simulink model "MatlabDDE"  (Simulink 7.3)
settings: Solver=ode3  StartTime=0.0  StopTime=inf  FixedStep=0.1  RelTol=1e-3
libraries: ddelib x10
settings Model: Creator=Marcin  LastModifiedBy=Marcin  ExtModeBatchMode=on  BufferReuse=off
settings DataIOCC: SaveOutput=off  SaveTime=off
settings OptimizationCC: BlockReduction=off  ConditionallyExecuteInputs=off  OptimizeBlockIOStorage=off  BufferReuse=off  ExpressionFolding=off  EnableMemcpy=off  FoldNonRolledExpr=off  LocalBlockOutputs=off  EfficientMapNaN2IntZero=off
settings RTWCC: GenerateMakefile=off  GenerateReport=on  RetainRTWFile=on  ProcessScript=grt_make_rtw_hook  LaunchReport=on  TargetLang=C++  RTWCompilerOptimization=On
settings CodeAppCC: ForceParamTrailComments=on

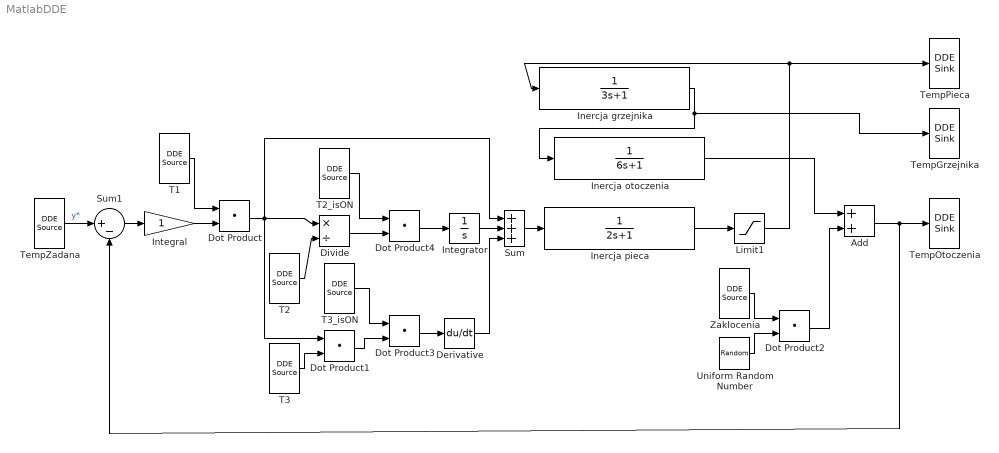
== system MatlabDDE ==
  Add : Sum  OutDataType=fixdt(1, 16)  OutScaling=2^-10
  Derivative : Derivative
  Divide : Product  Inputs=*/  OutDataType=fixdt(1, 16)  OutScaling=2^-10
  Dot Product{,1..4} (5 alike) : DotProduct  OutDataType=fixdt(1, 16)  OutScaling=2^-10  InputSameDT=on  OutDataTypeStr=Inherit: Inherit via internal rule
  Inercja grzejnika : TransferFcn  Denominator=[3 1]
  Inercja otoczenia : TransferFcn  Denominator=[6 1]
  Inercja pieca : TransferFcn  Denominator=[2 1]
  Integral : Gain  ParameterDataType=sfix(16)  ParameterScaling=2^0  OutDataType=sfix(16)  OutScaling=2^0  SaturateOnIntegerOverflow=on  OutDataTypeStr=Inherit: Same as input  ParamDataTypeStr=Inherit: Same as input
  Integrator : Integrator
  Limit1 : Saturate  UpperLimit=100  LowerLimit=0  OutDataType=fixdt(1, 16)  OutScaling=2^0
  Sum : Sum  Inputs=+++  OutDataType=sfix(16)  OutScaling=2^0  SaturateOnIntegerOverflow=on  InputSameDT=on  OutDataTypeStr=Inherit: Same as first input
  Sum1 : Sum  Inputs=|+-  OutDataType=sfix(16)  OutScaling=2^0  SaturateOnIntegerOverflow=on
  T1 : ddelib/DDE Source  SystemSampleTime=-1  service='view'  topic='tagname'  item='T1'
  T2 : ddelib/DDE Source  SystemSampleTime=-1  service='view'  topic='tagname'  item='T2'
  T2_isON : ddelib/DDE Source  SystemSampleTime=-1  service='view'  topic='tagname'  item='T2_isON'
  T3 : ddelib/DDE Source  SystemSampleTime=-1  service='view'  topic='tagname'  item='T3'
  T3_isON : ddelib/DDE Source  SystemSampleTime=-1  service='view'  topic='tagname'  item='T3_isOn'
  TempGrzejnika : ddelib/DDE Sink  SystemSampleTime=-1  service='view'  topic='tagname'  item='TempGrzejnika'
  TempOtoczenia : ddelib/DDE Sink  SystemSampleTime=-1  service='view'  topic='tagname'  item='TempOtoczenia'
  TempPieca : ddelib/DDE Sink  SystemSampleTime=-1  service='view'  topic='tagname'  item='TempPieca'
  TempZadana : ddelib/DDE Source  SystemSampleTime=-1  service='view'  topic='tagname'  item='TempZadanaOtoczenia'
  Uniform Random Number : UniformRandomNumber  SampleTime=0.1
  Zaklocenia : ddelib/DDE Source  SystemSampleTime=-1  service='view'  topic='tagname'  item='Straty'
  wires:
  Integrator/1 -> Sum/2
  Sum/1 -> Inercja pieca/1
  T3/1 -> Dot Product1/2
  T1/1 -> Dot Product/1
  Sum1/1 -> Integral/1
  Dot Product/1 -> Divide/1, Dot Product1/1, Sum/1
  T2/1 -> Divide/2
  Integral/1 -> Dot Product/2
  Derivative/1 -> Sum/3
  TempZadana/1 -> Sum1/1  "y*"
  Add/1 -> TempOtoczenia/1, Sum1/2
  Inercja otoczenia/1 -> Add/1
  Inercja pieca/1 -> Limit1/1
  Limit1/1 -> Inercja grzejnika/1, TempPieca/1
  Zaklocenia/1 -> Dot Product2/1
  Uniform Random Number/1 -> Dot Product2/2
  Dot Product2/1 -> Add/2
  Dot Product3/1 -> Derivative/1
  Dot Product1/1 -> Dot Product3/2
  T3_isON/1 -> Dot Product3/1
  Dot Product4/1 -> Integrator/1
  Divide/1 -> Dot Product4/2
  T2_isON/1 -> Dot Product4/1
  Inercja grzejnika/1 -> Inercja otoczenia/1, TempGrzejnika/1
